simulink model "PS8_tank_modified_D_acting_on_y"  (R2015b)
settings: Solver=VariableStepAuto  StartTime=0.0  StopTime=300  RelTol=1e-3
undefined symbols (not defined in the file or in its folder): G_PID_PAR, tank_pid_mod
settings Model: Creator=kjartan  LastModifiedBy=kjartan

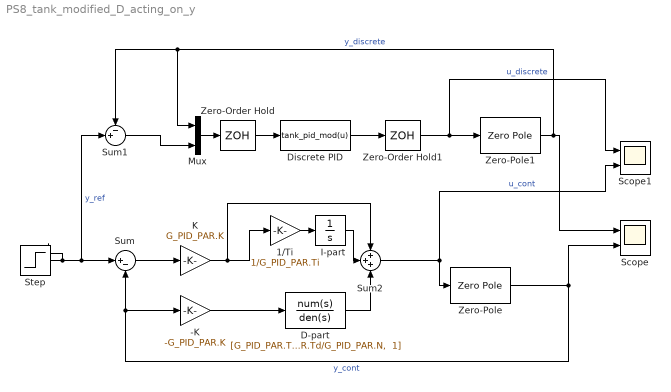
== system PS8_tank_modified_D_acting_on_y ==
  -K : Gain  Gain=-G_PID_PAR.K
  1/Ti : Gain  Gain=1/G_PID_PAR.Ti
  D-part : TransferFcn  Numerator=[G_PID_PAR.Td, 0]  Denominator="[G_PID_PAR.Td/G_PID_PAR.N,  1]"
  Discrete PID : MATLABFcn  MATLABFcn=tank_pid_mod(u)  OutputDimensions=1  Output1D=off
  I-part : Integrator
  K : Gain  Gain=G_PID_PAR.K
  Mux : Mux  Inputs=2
  Scope : Scope  NumInputPorts=2
  Scope1 : Scope  NumInputPorts=2
  Step : Step  SampleTime=0
  Sum : Sum  Inputs=|+-
  Sum1 : Sum  Inputs=-+|
  Sum2 : Sum  Inputs=+++
  Zero-Order Hold : ZeroOrderHold  SampleTime=G_PID_PAR.h
  Zero-Order Hold1 : ZeroOrderHold  SampleTime=G_PID_PAR.h
  Zero-Pole : ZeroPole  Zeros=[]  Poles=[-0.0179, -0.0129]  Gain=[0.00048]
  Zero-Pole1 : ZeroPole  Zeros=[]  Poles=[-0.0179, -0.0129]  Gain=[0.00048]
  wires:
  Sum/1 -> K/1
  Zero-Pole/1 -> Scope/2, Sum/2, -K/1  "y_cont"
  Step/1 -> Sum1/2, Sum/1  "y_ref"
  Zero-Order Hold/1 -> Discrete PID/1
  Discrete PID/1 -> Zero-Order Hold1/1
  Zero-Order Hold1/1 -> Scope1/1, Zero-Pole1/1  "u_discrete"
  Sum2/1 -> Scope1/2, Zero-Pole/1  "u_cont"
  Zero-Pole1/1 -> Scope/1, Mux/1, Sum1/1  "y_discrete"
  K/1 -> 1/Ti/1, Sum2/1
  I-part/1 -> Sum2/2
  D-part/1 -> Sum2/3
  1/Ti/1 -> I-part/1
  Sum1/1 -> Mux/2
  Mux/1 -> Zero-Order Hold/1
  -K/1 -> D-part/1
